simulink model "pendulum"  (R2022a)
settings: Solver=ode1  StartTime=0.0  StopTime=10.0  FixedStep=1/50  RelTol=1e-3
PostLoadFcn:
  | src_path = fullfile(fileparts(which(bdroot)),'..')
  | run(fullfile(src_path, 'code', 'callbacks','init_pendulum.m'))
undefined symbols (not defined in the file): control, plant
settings Model: Creator=enrique.babio  LastModifiedBy=enrique.babio
settings DataIOCC: SaveFinalState=on  SaveState=on  DSMLogging=off  InspectSignalLogs=on  ReturnWorkspaceOutputsName=simout

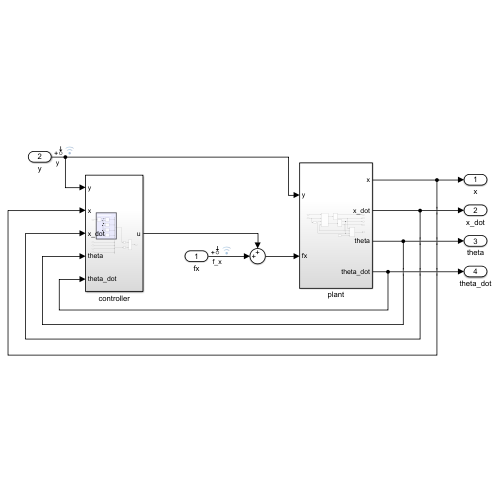
[thumbnail: Simulink's stored preview of the top-level diagram]
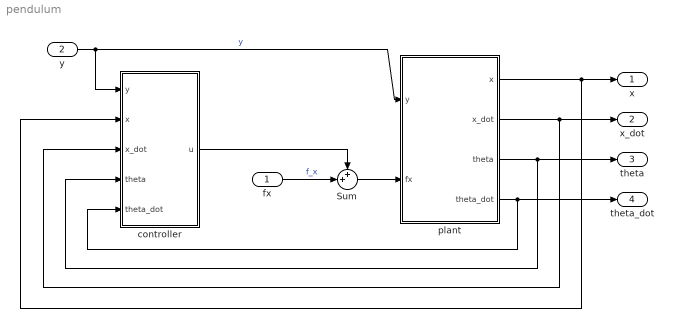
== system pendulum ==
  fx : Inport  Interpolate=off
  y : Inport  Port=2  Interpolate=off
  Sum : Sum  Inputs=++|
  controller : Subsystem
  plant : Subsystem
  x : Outport
  x_dot : Outport  Port=2
  theta : Outport  Port=3
  theta_dot : Outport  Port=4
  wires:
  y/1 -> controller/1(y), plant/1(y)  "y"
  plant/1(x) -> x/1, controller/2(x)
  plant/2(x_dot) -> x_dot/1, controller/3(x_dot)
  plant/3(theta) -> theta/1, controller/4(theta)
  plant/4(theta_dot) -> controller/5(theta_dot), theta_dot/1
  Sum/1 -> plant/2(fx)
  fx/1 -> Sum/2  "f_x"
  controller/1(u) -> Sum/1

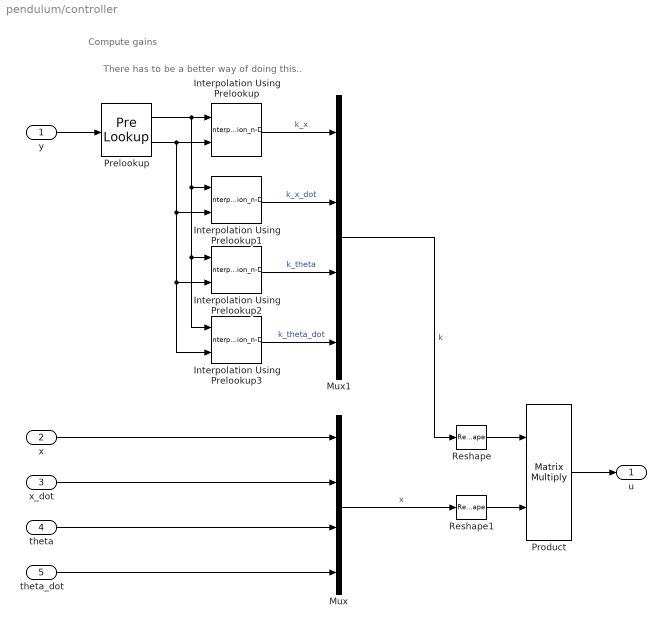
== system pendulum/controller ==
  note: There has to be a better way of doing this..
  note: Compute gains
  y : Inport
  x : Inport  Port=2
  x_dot : Inport  Port=3
  theta : Inport  Port=4
  theta_dot : Inport  Port=5
  Interpolation Using Prelookup : Interpolation_n-D  NumberOfTableDimensions=1  Table=squeeze(control.k(:,1,:))  InternalRulePriority=Speed
      settings: InputPortMap=u0,u1
  Interpolation Using Prelookup1 : Interpolation_n-D  NumberOfTableDimensions=1  Table=squeeze(control.k(:,2,:))  InternalRulePriority=Speed
      settings: InputPortMap=u0,u1
  Interpolation Using Prelookup2 : Interpolation_n-D  NumberOfTableDimensions=1  Table=squeeze(control.k(:,3,:))  InternalRulePriority=Speed
      settings: InputPortMap=u0,u1
  Interpolation Using Prelookup3 : Interpolation_n-D  NumberOfTableDimensions=1  Table=squeeze(control.k(:,4,:))  InternalRulePriority=Speed
      settings: InputPortMap=u0,u1
  Mux : Mux
  Mux1 : Mux
  Prelookup : PreLookup  BreakpointsData=control.y_scheduling  IndexSearchMethod=Linear search  BeginIndexSearchUsingPreviousIndexResult=on  ExtrapMethod=Linear
  Product : Product  Multiplication=Matrix(*)
  Reshape : Reshape  OutputDimensionality=Row vector (2-D)
  Reshape1 : Reshape  OutputDimensionality=Column vector (2-D)
  u : Outport
  wires:
  Mux/1 -> Reshape1/1  "x"
  x/1 -> Mux/1
  theta/1 -> Mux/3
  Product/1 -> u/1
  x_dot/1 -> Mux/2
  theta_dot/1 -> Mux/4
  y/1 -> Prelookup/1
  Prelookup/1 -> Interpolation Using Prelookup3/1, Interpolation Using Prelookup2/1, Interpolation Using Prelookup1/1, Interpolation Using Prelookup/1
  Prelookup/2 -> Interpolation Using Prelookup3/2, Interpolation Using Prelookup2/2, Interpolation Using Prelookup1/2, Interpolation Using Prelookup/2
  Interpolation Using Prelookup/1 -> Mux1/1  "k_x"
  Interpolation Using Prelookup1/1 -> Mux1/2  "k_x_dot"
  Interpolation Using Prelookup2/1 -> Mux1/3  "k_theta"
  Interpolation Using Prelookup3/1 -> Mux1/4  "k_theta_dot"
  Mux1/1 -> Reshape/1  "k"
  Reshape/1 -> Product/1
  Reshape1/1 -> Product/2

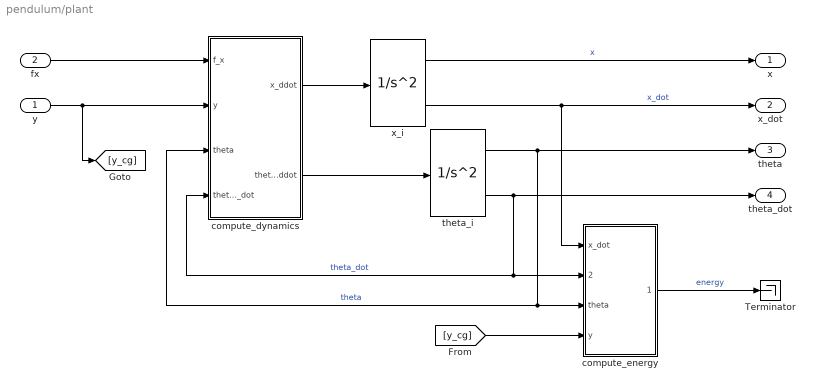
== system pendulum/plant ==
  y : Inport  Interpolate=off
  fx : Inport  Port=2  Interpolate=off
  Terminator : Terminator
  compute_dynamics : Subsystem
  compute_energy : Subsystem
  theta_i : SecondOrderIntegrator  ICX=0  WrapX=on  WrappedUpperValueX=pi/2  WrappedLowerValueX=-3/2*pi  StateNameX='theta'  ICDXDT=0  StateNameDXDT='theta_dot'  ZeroCross=off
  x_i : SecondOrderIntegrator  StateNameX='x'  ICDXDT=0  StateNameDXDT='x_dot'  ZeroCross=off
  x : Outport
  x_dot : Outport  Port=2
  theta : Outport  Port=3
  theta_dot : Outport  Port=4
  wires:
  fx/1 -> compute_dynamics/1(f_x)
  y/1 -> [y_cg], compute_dynamics/2(y)
  theta_i/1 -> theta/1, compute_dynamics/3(theta), compute_energy/3(theta)  "theta"
  theta_i/2 -> theta_dot/1, compute_dynamics/4(theta_dot), compute_energy/2(theta_ddot)  "theta_dot"
  x_i/2 -> x_dot/1, compute_energy/1(x_dot)  "x_dot"
  compute_dynamics/2(theta_ddot) -> theta_i/1
  compute_energy/1(energy) -> Terminator/1  "energy"
  [y_cg] -> compute_energy/4(y)
  compute_dynamics/1(x_ddot) -> x_i/1
  x_i/1 -> x/1  "x"

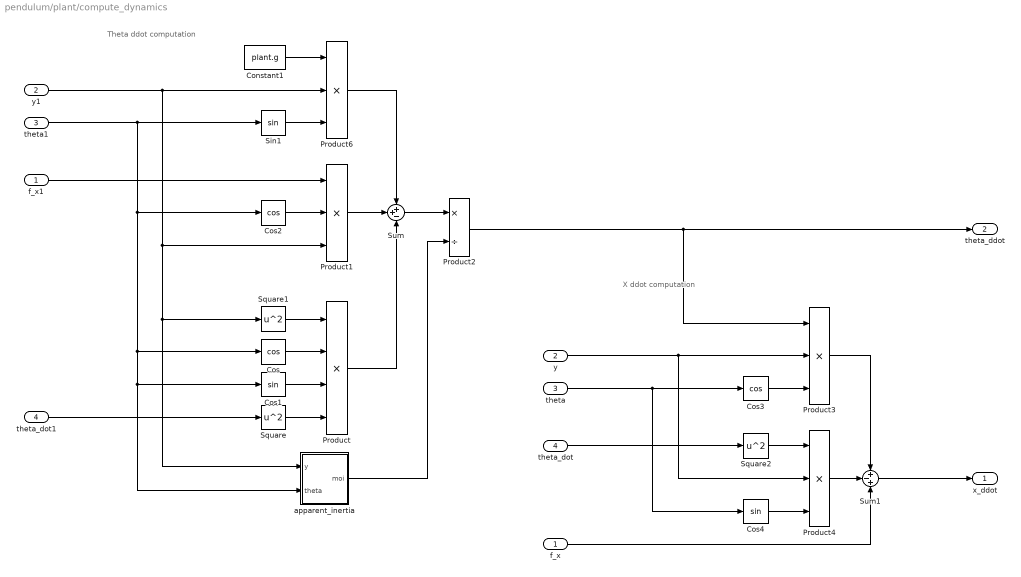
== system pendulum/plant/compute_dynamics ==
  note: X ddot computation
  note: Theta ddot computation
  f_x : Inport
  y : Inport  Port=2
  theta : Inport  Port=3
  theta_dot : Inport  Port=4
  Constant1 : Constant  Value=plant.g
  Cos : Trigonometry  Operator=cos
  Cos1 : Trigonometry
  Cos2 : Trigonometry  Operator=cos
  Cos3 : Trigonometry  Operator=cos
  Cos4 : Trigonometry
  Product : Product  Inputs=4
  Product{1,3..4,6} (4 alike) : Product  Inputs=3
  Product2 : Product  Inputs=*/
  Sin1 : Trigonometry
  Square : Math  Operator=square
  Square1 : Math  Operator=square
  Square2 : Math  Operator=square
  Sum : Sum  Inputs=++-
  Sum1 : Sum  Inputs=+-+
  apparent_inertia : Subsystem
  f_x1 : InportShadow
  theta1 : InportShadow  Port=3
  theta_dot1 : InportShadow  Port=4
  y1 : InportShadow  Port=2
  x_ddot : Outport
  theta_ddot : Outport  Port=2
  wires:
  theta/1 -> Cos4/1, Cos3/1
  Cos1/1 -> Product/3
  y/1 -> Product4/2, Product3/2
  Product/1 -> Sum/3
  theta_dot/1 -> Square2/1
  Square1/1 -> Product/1
  Square/1 -> Product/4
  Product6/1 -> Sum/1
  Product1/1 -> Sum/2
  Sin1/1 -> Product6/3
  Cos/1 -> Product/2
  apparent_inertia/1(moi) -> Product2/2
  Sum/1 -> Product2/1
  Product2/1 -> Product3/1, theta_ddot/1
  Cos2/1 -> Product1/2
  Square2/1 -> Product4/1
  theta_dot1/1 -> Square/1
  theta1/1 -> apparent_inertia/2(theta), Cos1/1, Cos/1, Cos2/1, Sin1/1
  f_x1/1 -> Product1/1
  Cos4/1 -> Product4/3
  Sum1/1 -> x_ddot/1
  y1/1 -> Product6/2, apparent_inertia/1(y), Square1/1, Product1/3
  Constant1/1 -> Product6/1
  Cos3/1 -> Product3/3
  Product4/1 -> Sum1/2
  f_x/1 -> Sum1/3
  Product3/1 -> Sum1/1

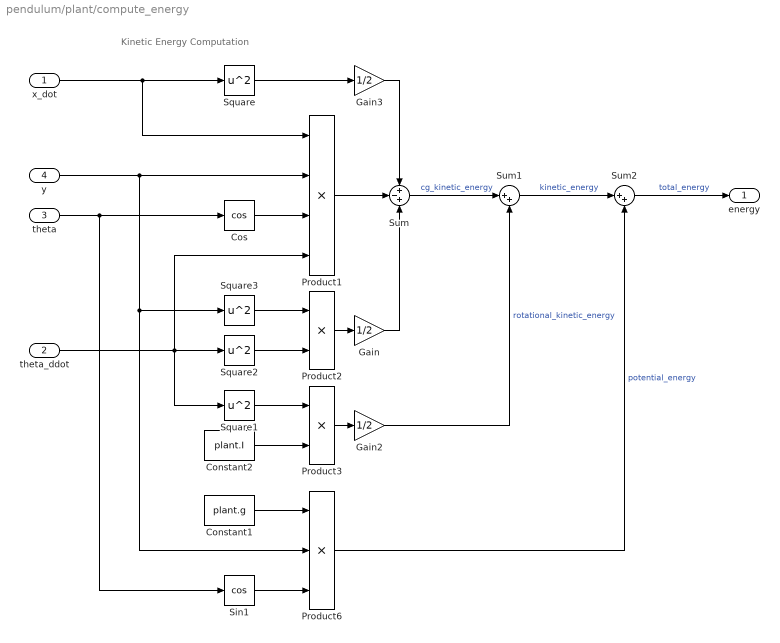
== system pendulum/plant/compute_energy ==
  note: Kinetic Energy Computation
  x_dot : Inport
  theta_ddot : Inport  Port=2
  theta : Inport  Port=3
  y : Inport  Port=4
  Constant1 : Constant  Value=plant.g
  Constant2 : Constant  Value=plant.I
  Cos : Trigonometry  Operator=cos
  Gain : Gain  Gain=1/2
  Gain2 : Gain  Gain=1/2
  Gain3 : Gain  Gain=1/2
  Product1 : Product  Inputs=4
  Product2 : Product
  Product3 : Product
  Product6 : Product  Inputs=3
  Sin1 : Trigonometry  Operator=cos
  Square{,1..3} (4 alike) : Math  Operator=square
  Sum : Sum  Inputs=+-+
  Sum1 : Sum  Inputs=|++
  Sum2 : Sum  Inputs=|++
  energy : Outport
  wires:
  theta_ddot/1 -> Square1/1, Product1/4, Square2/1
  x_dot/1 -> Square/1, Product1/1
  Product1/1 -> Sum/2
  Product2/1 -> Gain/1
  Square/1 -> Gain3/1
  Cos/1 -> Product1/3
  Square2/1 -> Product2/2
  Square3/1 -> Product2/1
  Square1/1 -> Product3/1
  Product3/1 -> Gain2/1
  Sum1/1 -> Sum2/1  "kinetic_energy"
  Sum2/1 -> energy/1  "total_energy"
  Product6/1 -> Sum2/2  "potential_energy"
  Gain2/1 -> Sum1/2  "rotational_kinetic_energy"
  Sum/1 -> Sum1/1  "cg_kinetic_energy"
  Gain/1 -> Sum/3
  Gain3/1 -> Sum/1
  Constant1/1 -> Product6/1
  Sin1/1 -> Product6/3
  theta/1 -> Sin1/1, Cos/1
  y/1 -> Product1/2, Product6/2, Square3/1
  Constant2/1 -> Product3/2

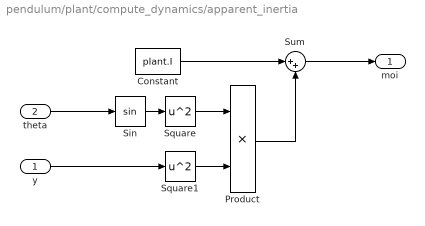
== system pendulum/plant/compute_dynamics/apparent_inertia ==
  y : Inport
  theta : Inport  Port=2
  Constant : Constant  Value=plant.I
  Product : Product
  Sin : Trigonometry
  Square : Math  Operator=square
  Square1 : Math  Operator=square
  Sum : Sum  Inputs=|++
  moi : Outport
  wires:
  Square/1 -> Product/1
  Product/1 -> Sum/2
  Constant/1 -> Sum/1
  y/1 -> Square1/1
  Sin/1 -> Square/1
  Sum/1 -> moi/1
  theta/1 -> Sin/1
  Square1/1 -> Product/2
